simulink model "HCS_Sim_r9_final"  (R2023a)
settings: Solver=ode4  StartTime=0.0  StopTime=24  FixedStep=5e-3  RelTol=1e-3  EnableMultiTasking=on
libraries: simulink x26, simulink_extras x11, arduinolib x8, spspowerguiLib x1
(part 4 of 5)

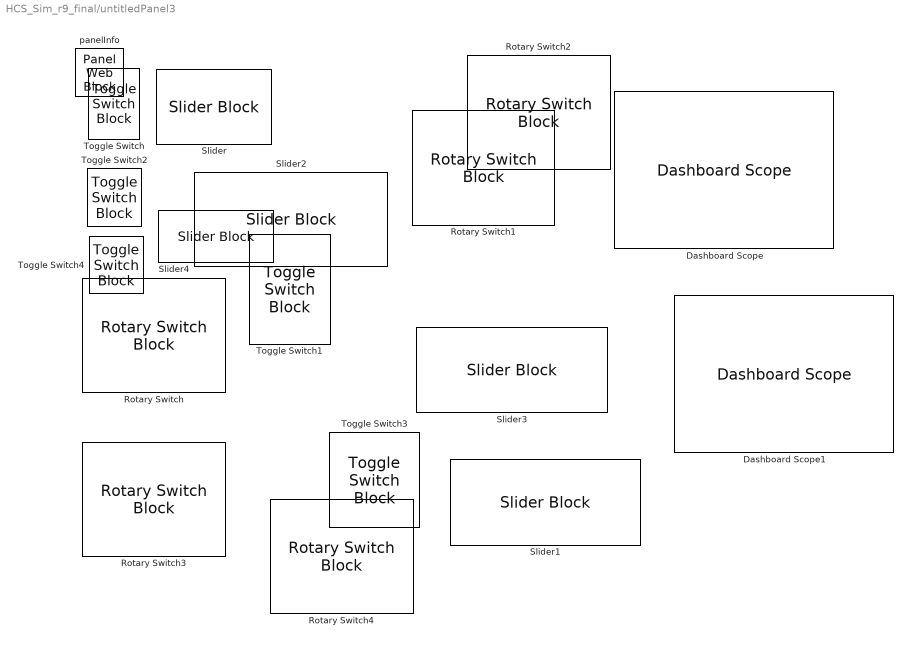
== system HCS_Sim_r9_final/untitledPanel3 ==
  Dashboard Scope : DashboardScope  Tag=HiddenForWebPanel  PanelInfo="{\"height\":377,\"left\":709,\"panelId\":\"panelId-5b2835c8-b6db-4cff-a750-dd4ee5f35628\",\"top\":424,\"type\":\"panelChild\",\"version\":\"2019b\",\"width\":535,\"zIndex\":1500032}"
  Dashboard Scope1 : DashboardScope  Tag=HiddenForWebPanel  PanelInfo="{\"height\":385,\"left\":705,\"panelId\":\"panelId-5b2835c8-b6db-4cff-a750-dd4ee5f35628\",\"top\":16,\"type\":\"panelChild\",\"version\":\"2019b\",\"width\":524,\"zIndex\":1500034}"
  Rotary Switch : RotarySwitchBlock  Tag=HiddenForWebPanel  PanelInfo="{\"height\":145,\"left\":20,\"panelId\":\"panelId-5b2835c8-b6db-4cff-a750-dd4ee5f35628\",\"top\":16,\"type\":\"panelChild\",\"version\":\"2019b\",\"width\":182,\"zIndex\":1500016}"
      settings: Values={{'>0', '1', '2', '3', '4'}, [0 1 2 3 4]}
      settings: AttributesFormatString=Hydrogren Level
  Rotary Switch1 : RotarySwitchBlock  Tag=HiddenForWebPanel  PanelInfo="{\"height\":145,\"left\":24,\"panelId\":\"panelId-5b2835c8-b6db-4cff-a750-dd4ee5f35628\",\"top\":177,\"type\":\"panelChild\",\"version\":\"2019b\",\"width\":182,\"zIndex\":1500014}"
      settings: Values={{'>0', '1', '2', '3', '4'}, [0 1 2 3 4]}
      settings: AttributesFormatString=Hydrogren Level
  Rotary Switch2 : RotarySwitchBlock  Tag=HiddenForWebPanel  PanelInfo="{\"height\":145,\"left\":24,\"panelId\":\"panelId-5b2835c8-b6db-4cff-a750-dd4ee5f35628\",\"top\":334,\"type\":\"panelChild\",\"version\":\"2019b\",\"width\":182,\"zIndex\":1500018}"
      settings: Values={{'>0', '1', '2', '3', '4'}, [0 1 2 3 4]}
      settings: AttributesFormatString=Hydrogren Level
  Rotary Switch3 : RotarySwitchBlock  Tag=HiddenForWebPanel  PanelInfo="{\"height\":145,\"left\":26,\"panelId\":\"panelId-5b2835c8-b6db-4cff-a750-dd4ee5f35628\",\"top\":492,\"type\":\"panelChild\",\"version\":\"2019b\",\"width\":182,\"zIndex\":1500020}"
      settings: Values={{'>0', '1', '2', '3', '4'}, [0 1 2 3 4]}
      settings: AttributesFormatString=Hydrogren Level
  Rotary Switch4 : RotarySwitchBlock  Tag=HiddenForWebPanel  PanelInfo="{\"height\":145,\"left\":33,\"panelId\":\"panelId-5b2835c8-b6db-4cff-a750-dd4ee5f35628\",\"top\":649,\"type\":\"panelChild\",\"version\":\"2019b\",\"width\":182,\"zIndex\":1500022}"
      settings: Values={{'>0', '1', '2', '3', '4'}, [0 1 2 3 4]}
      settings: AttributesFormatString=Hydrogren Level
  Slider : SliderBlock  Tag=HiddenForWebPanel  PanelInfo="{\"height\":135,\"left\":211,\"panelId\":\"panelId-5b2835c8-b6db-4cff-a750-dd4ee5f35628\",\"top\":22,\"type\":\"panelChild\",\"version\":\"2019b\",\"width\":253,\"zIndex\":1500008}"  ScaleMax=24
      settings: AttributesFormatString=Start Time
  Slider1 : SliderBlock  Tag=HiddenForWebPanel  PanelInfo="{\"height\":145,\"left\":217,\"panelId\":\"panelId-5b2835c8-b6db-4cff-a750-dd4ee5f35628\",\"top\":492,\"type\":\"panelChild\",\"version\":\"2019b\",\"width\":247,\"zIndex\":1500026}"  ScaleMax=24
      settings: AttributesFormatString=Start Time
  Slider2 : SliderBlock  Tag=HiddenForWebPanel  PanelInfo="{\"height\":145,\"left\":215,\"panelId\":\"panelId-5b2835c8-b6db-4cff-a750-dd4ee5f35628\",\"top\":177,\"type\":\"panelChild\",\"version\":\"2019b\",\"width\":236,\"zIndex\":1500036}"  ScaleMax=24  TickInterval=3
  Slider3 : SliderBlock  Tag=HiddenForWebPanel  PanelInfo="{\"height\":137,\"left\":217,\"panelId\":\"panelId-5b2835c8-b6db-4cff-a750-dd4ee5f35628\",\"top\":336,\"type\":\"panelChild\",\"version\":\"2019b\",\"width\":241,\"zIndex\":1500024}"  ScaleMax=24
      settings: AttributesFormatString=Start Time
  Slider4 : SliderBlock  Tag=HiddenForWebPanel  PanelInfo="{\"height\":133,\"left\":227,\"panelId\":\"panelId-5b2835c8-b6db-4cff-a750-dd4ee5f35628\",\"top\":654,\"type\":\"panelChild\",\"version\":\"2019b\",\"width\":242,\"zIndex\":1500012}"  ScaleMax=24
      settings: AttributesFormatString=Start Time
  Toggle Switch : ToggleSwitchBlock  Tag=HiddenForWebPanel  PanelInfo="{\"height\":140,\"left\":472,\"panelId\":\"panelId-5b2835c8-b6db-4cff-a750-dd4ee5f35628\",\"top\":11,\"type\":\"panelChild\",\"version\":\"2019b\",\"width\":131,\"zIndex\":1500002}"
      settings: Values={{'Off', 'On'}, [0 1]}
  Toggle Switch1 : ToggleSwitchBlock  Tag=HiddenForWebPanel  PanelInfo="{\"height\":129,\"left\":473,\"panelId\":\"panelId-5b2835c8-b6db-4cff-a750-dd4ee5f35628\",\"top\":160,\"type\":\"panelChild\",\"version\":\"2019b\",\"width\":130,\"zIndex\":1500028}"
      settings: Values={{'Off', 'On'}, [0 1]}
  Toggle Switch2 : ToggleSwitchBlock  Tag=HiddenForWebPanel  PanelInfo="{\"height\":142,\"left\":479,\"panelId\":\"panelId-5b2835c8-b6db-4cff-a750-dd4ee5f35628\",\"top\":468,\"type\":\"panelChild\",\"version\":\"2019b\",\"width\":133,\"zIndex\":1500004}"
      settings: Values={{'Off', 'On'}, [0 1]}
  Toggle Switch3 : ToggleSwitchBlock  Tag=HiddenForWebPanel  PanelInfo="{\"height\":155,\"left\":483,\"panelId\":\"panelId-5b2835c8-b6db-4cff-a750-dd4ee5f35628\",\"top\":624,\"type\":\"panelChild\",\"version\":\"2019b\",\"width\":140,\"zIndex\":1500030}"
      settings: Values={{'Off', 'On'}, [0 1]}
  Toggle Switch4 : ToggleSwitchBlock  Tag=HiddenForWebPanel  PanelInfo="{\"height\":148,\"left\":479,\"panelId\":\"panelId-5b2835c8-b6db-4cff-a750-dd4ee5f35628\",\"top\":301,\"type\":\"panelChild\",\"version\":\"2019b\",\"width\":126,\"zIndex\":1500006}"
      settings: Values={{'Off', 'On'}, [0 1]}
  panelInfo : PanelWebBlock  Tag=HiddenForWebPanel  PanelInfo="{\"compacted\":false,\"height\":812,\"isActiveTab\":true,\"left\":344,\"name\":\"Panel3\",\"panelId\":\"panelId-5b2835c8-b6db-4cff-a750-dd4ee5f35628\",\"tabIndex\":3,\"tabbedSetId\":\"tabbedSet1419519353\",\"top\":42,\"type\":\"panel\",\"version\":\"2019b\",\"visible\":true,\"width\":1334,\"zIndex\":1500006}"  PanelSnapshot=<binary blob, 125788 chars, not shown>  PanelBackground=data:image/png;base64,iVBORw0KGgoAAAANSUhEUgAAA9QAAAJiCAYAAAAmMIpYAAAAAXNSR0IArs4c6QAAAARnQU1BAACxjwv8YQUAAAAJcEhZcwAADsQAAA7EAZUrDhsAAE72SURBVHhe7d15tGZ5WR/636nh1Fw9NyBiCyIqaLyAEUQUUa8iOCBOBMc4haiEqwQ14sq9ioBTdCUKLr1CEgeUdRMjiDgQBQ0GEwcUBJRWBJFOC/RQ46mqU+fU/X33fp9zdr+eBtxBu4bPZ62nf8Pe73Tgn289+93vyoWuAQAAAH8nuxYjAAAA8HcgUAMAAMAMAjUAAADMIFADAADADAI1AAAAzCBQAwAAwAwCNQAAAMwgUAMAAMAMAjUAAADMIFADAADADAI1AAAAzCBQAwAAwAwCNQAA ...(+26696 chars)

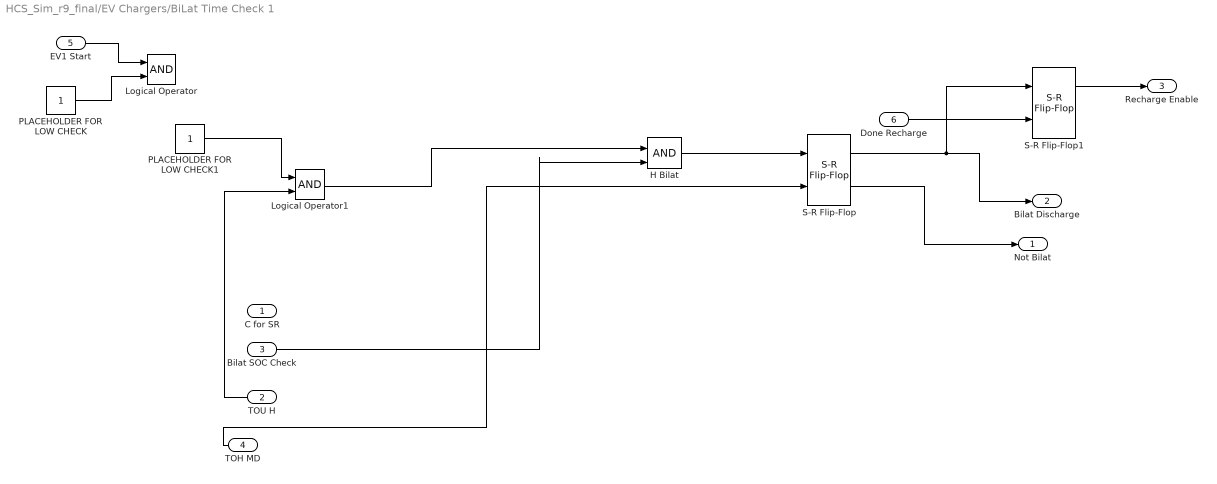
== system HCS_Sim_r9_final/EV Chargers/BiLat Time Check 1 ==
  C for SR : Inport
  TOU H : Inport  Port=2
  Bilat SOC Check : Inport  Port=3
  TOH MD : Inport  Port=4
  EV1 Start : Inport  Port=5
  Done Recharge : Inport  Port=6
  H Bilat : Logic  IconShape=distinctive  AllPortsSameDT=off  OutDataTypeStr=boolean
  Logical Operator : Logic  AllPortsSameDT=off  OutDataTypeStr=boolean
  Logical Operator1 : Logic  AllPortsSameDT=off  OutDataTypeStr=boolean
  PLACEHOLDER FOR LOW CHECK : Constant
  PLACEHOLDER FOR LOW CHECK1 : Constant
  S-R Flip-Flop : simulink_extras/Flip Flops/S-R Flip-Flop  initial_condition=0
  S-R Flip-Flop1 : simulink_extras/Flip Flops/S-R Flip-Flop  initial_condition=0
  Not Bilat : Outport
  Bilat Discharge : Outport  Port=2
  Recharge Enable : Outport  Port=3
  wires:
  TOH MD/1 -> S-R Flip-Flop/2
  Logical Operator1/1 -> H Bilat/1
  PLACEHOLDER FOR LOW CHECK1/1 -> Logical Operator1/1
  H Bilat/1 -> S-R Flip-Flop/1
  S-R Flip-Flop/1 -> S-R Flip-Flop1/1, Bilat Discharge/1
  S-R Flip-Flop/2 -> Not Bilat/1
  Bilat SOC Check/1 -> H Bilat/2
  TOU H/1 -> Logical Operator1/2
  PLACEHOLDER FOR LOW CHECK/1 -> Logical Operator/2
  EV1 Start/1 -> Logical Operator/1
  S-R Flip-Flop1/1 -> Recharge Enable/1
  Done Recharge/1 -> S-R Flip-Flop1/2

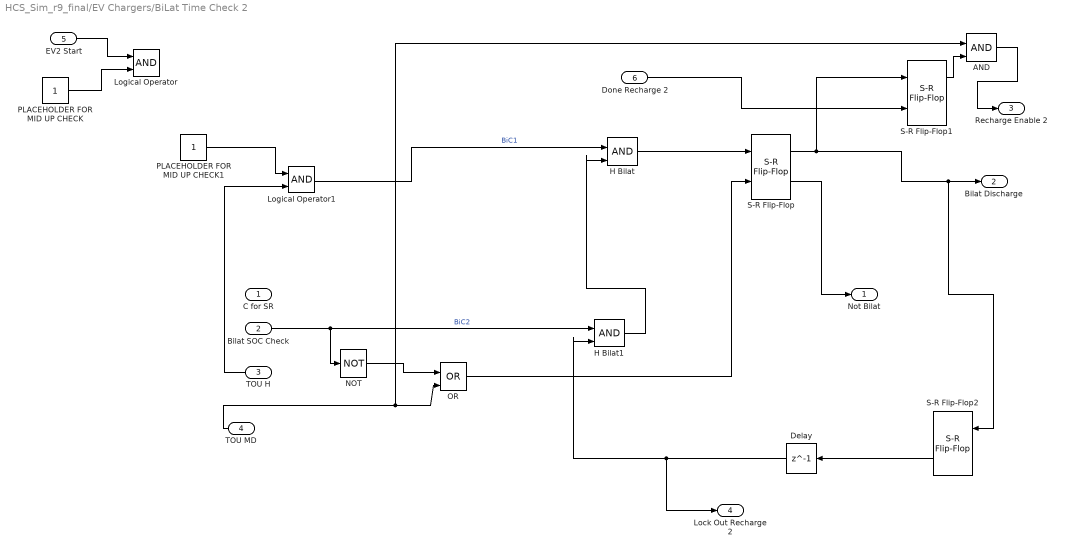
== system HCS_Sim_r9_final/EV Chargers/BiLat Time Check 2 ==
  C for SR : Inport
  Bilat SOC Check : Inport  Port=2
  TOU H : Inport  Port=3
  TOU MD : Inport  Port=4
  EV2 Start : Inport  Port=5
  Done Recharge 2 : Inport  Port=6
  AND : Logic  IconShape=distinctive  AllPortsSameDT=off  OutDataTypeStr=boolean
  Delay : Delay  DelayLength=1  InitialCondition=0
  H Bilat : Logic  IconShape=distinctive  AllPortsSameDT=off  OutDataTypeStr=boolean
  H Bilat1 : Logic  IconShape=distinctive  AllPortsSameDT=off  OutDataTypeStr=boolean
  Logical Operator : Logic  AllPortsSameDT=off  OutDataTypeStr=boolean
  Logical Operator1 : Logic  AllPortsSameDT=off  OutDataTypeStr=boolean
  NOT : Logic  Operator=NOT  IconShape=distinctive  AllPortsSameDT=off  OutDataTypeStr=boolean
  OR : Logic  Operator=OR  IconShape=distinctive  AllPortsSameDT=off  OutDataTypeStr=boolean
  PLACEHOLDER FOR MID UP CHECK : Constant
  PLACEHOLDER FOR MID UP CHECK1 : Constant
  S-R Flip-Flop : simulink_extras/Flip Flops/S-R Flip-Flop  initial_condition=0
  S-R Flip-Flop1 : simulink_extras/Flip Flops/S-R Flip-Flop  initial_condition=0
  S-R Flip-Flop2 : simulink_extras/Flip Flops/S-R Flip-Flop  initial_condition=0
  Not Bilat : Outport
  Bilat Discharge : Outport  Port=2
  Recharge Enable 2 : Outport  Port=3
  Lock Out Recharge 2 : Outport  Port=4
  wires:
  Logical Operator1/1 -> H Bilat/1  "BiC1"
  PLACEHOLDER FOR MID UP CHECK1/1 -> Logical Operator1/1
  S-R Flip-Flop/1 -> S-R Flip-Flop1/1, S-R Flip-Flop2/1, Bilat Discharge/1
  H Bilat/1 -> S-R Flip-Flop/1
  S-R Flip-Flop/2 -> Not Bilat/1
  Bilat SOC Check/1 -> H Bilat1/1, NOT/1  "BiC2"
  TOU H/1 -> Logical Operator1/2
  EV2 Start/1 -> Logical Operator/1
  PLACEHOLDER FOR MID UP CHECK/1 -> Logical Operator/2
  TOU MD/1 -> AND/1, OR/2
  Done Recharge 2/1 -> S-R Flip-Flop1/2
  AND/1 -> Recharge Enable 2/1
  OR/1 -> S-R Flip-Flop/2
  NOT/1 -> OR/1
  H Bilat1/1 -> H Bilat/2
  S-R Flip-Flop2/2 -> Delay/1
  Delay/1 -> Lock Out Recharge 2/1, H Bilat1/2
  S-R Flip-Flop1/1 -> AND/2

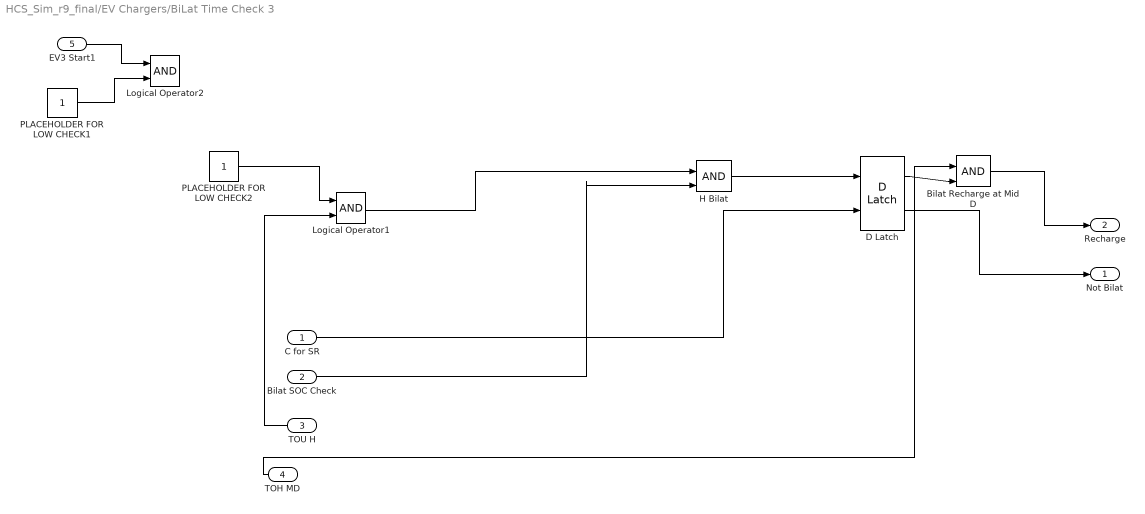
== system HCS_Sim_r9_final/EV Chargers/BiLat Time Check 3 ==
  C for SR : Inport
  Bilat SOC Check : Inport  Port=2
  TOU H : Inport  Port=3
  TOH MD : Inport  Port=4
  EV3 Start1 : Inport  Port=5
  Bilat Recharge at Mid D : Logic  IconShape=distinctive  AllPortsSameDT=off  OutDataTypeStr=boolean
  D Latch : simulink_extras/Flip Flops/D Latch
  H Bilat : Logic  IconShape=distinctive  AllPortsSameDT=off  OutDataTypeStr=boolean
  Logical Operator1 : Logic  AllPortsSameDT=off  OutDataTypeStr=boolean
  Logical Operator2 : Logic  AllPortsSameDT=off  OutDataTypeStr=boolean
  PLACEHOLDER FOR LOW CHECK1 : Constant
  PLACEHOLDER FOR LOW CHECK2 : Constant
  Not Bilat : Outport
  Recharge : Outport  Port=2
  wires:
  TOH MD/1 -> Bilat Recharge at Mid D/1
  Logical Operator1/1 -> H Bilat/1
  PLACEHOLDER FOR LOW CHECK2/1 -> Logical Operator1/1
  Bilat Recharge at Mid D/1 -> Recharge/1
  H Bilat/1 -> D Latch/1
  D Latch/1 -> Bilat Recharge at Mid D/2
  D Latch/2 -> Not Bilat/1
  C for SR/1 -> D Latch/2
  Bilat SOC Check/1 -> H Bilat/2
  TOU H/1 -> Logical Operator1/2
  EV3 Start1/1 -> Logical Operator2/1
  PLACEHOLDER FOR LOW CHECK1/1 -> Logical Operator2/2

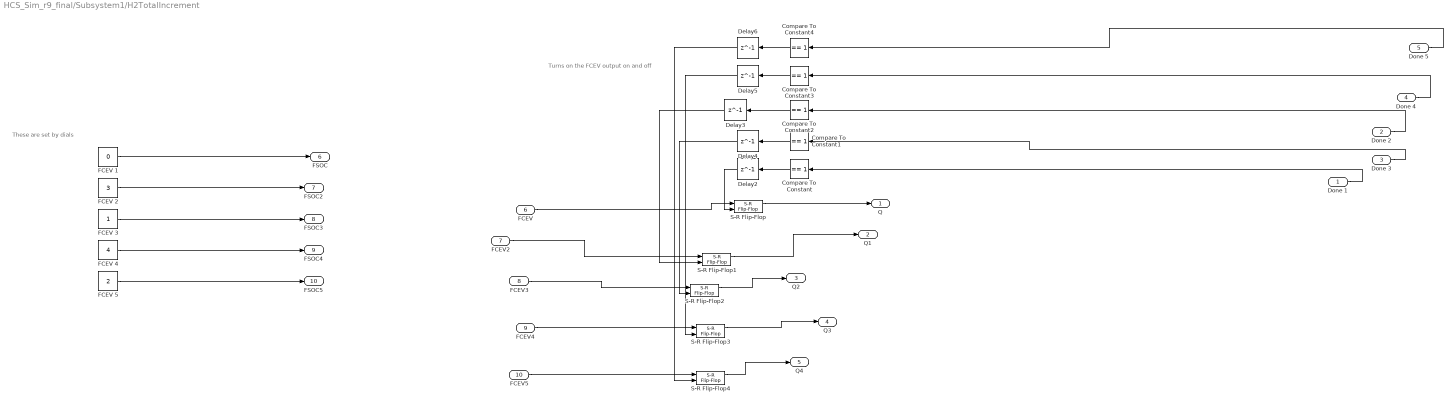
== system HCS_Sim_r9_final/Subsystem1/H2TotalIncrement ==
  note: Turns on the FCEV output
      | on and off
  note: These are set by dials
  Done 1 : Inport
  Done 2 : Inport  Port=2
  Done 3 : Inport  Port=3
  Done 4 : Inport  Port=4
  Done 5 : Inport  Port=5
  FCEV : Inport  Port=6
  FCEV2 : Inport  Port=7
  FCEV3 : Inport  Port=8
  FCEV4 : Inport  Port=9
  FCEV5 : Inport  Port=10
  Compare To Constant{,1..4} (5 alike) : simulink/Logic and Bit Operations/Compare To Constant  relop===  const=1  OutDataTypeStr=boolean
  Delay{2..6} (5 alike) : Delay  DelayLength=1  InitialCondition=0
  FCEV 1 : Constant  Value=0
  FCEV 2 : Constant  Value=3
  FCEV 3 : Constant
  FCEV 4 : Constant  Value=4
  FCEV 5 : Constant  Value=2
  S-R Flip-Flop{,1..4} (5 alike) : simulink_extras/Flip Flops/S-R Flip-Flop  initial_condition=0
  Q : Outport
  Q1 : Outport  Port=2
  Q2 : Outport  Port=3
  Q3 : Outport  Port=4
  Q4 : Outport  Port=5
  FSOC : Outport  Port=6
  FSOC2 : Outport  Port=7
  FSOC3 : Outport  Port=8
  FSOC4 : Outport  Port=9
  FSOC5 : Outport  Port=10
  wires:
  Done 5/1 -> Compare To Constant4/1
  Delay2/1 -> S-R Flip-Flop/2
  Delay4/1 -> S-R Flip-Flop2/2
  FCEV 3/1 -> FSOC3/1
  FCEV4/1 -> S-R Flip-Flop3/1
  FCEV 4/1 -> FSOC4/1
  Done 4/1 -> Compare To Constant3/1
  Delay6/1 -> S-R Flip-Flop4/2
  Compare To Constant4/1 -> Delay6/1
  Compare To Constant1/1 -> Delay4/1
  Compare To Constant3/1 -> Delay5/1
  Compare To Constant2/1 -> Delay3/1
  Compare To Constant/1 -> Delay2/1
  Delay3/1 -> S-R Flip-Flop1/2
  Delay5/1 -> S-R Flip-Flop3/2
  S-R Flip-Flop/1 -> Q/1
  S-R Flip-Flop4/1 -> Q4/1
  FCEV 5/1 -> FSOC5/1
  S-R Flip-Flop1/1 -> Q1/1
  FCEV5/1 -> S-R Flip-Flop4/1
  Done 1/1 -> Compare To Constant/1
  S-R Flip-Flop3/1 -> Q3/1
  Done 2/1 -> Compare To Constant2/1
  FCEV2/1 -> S-R Flip-Flop1/1
  S-R Flip-Flop2/1 -> Q2/1
  FCEV/1 -> S-R Flip-Flop/1
  FCEV 1/1 -> FSOC/1
  Done 3/1 -> Compare To Constant1/1
  FCEV 2/1 -> FSOC2/1
  FCEV3/1 -> S-R Flip-Flop2/1

== matlab function HCS_Sim_r9_final/EV Chargers/MATLAB Function1 ==
  data: ev1_bilat_OK output; ev2_bilat_OK output; ev3_bilat_OK output; soc_ev1 input; ev1_OK input; soc_ev2 input; ev2_OK input; soc_ev3 input; ev1_chargeBool output; ev2_chargeBool output; ev3_chargeBool output; ev3_OK input
  function [ev1_bilat_OK, ev2_bilat_OK, ev3_bilat_OK, ev1_chargeBool, ev2_chargeBool, ev3_chargeBool] = pctSOCCheck(soc_ev1, ev1_OK, soc_ev2, ev2_OK, soc_ev3, ev3_OK)
    bilatPartition = 90; % pct SOC
    fullCharge = 100; % pct SOC
    
    soc_ev_array = [soc_ev1, soc_ev2, soc_ev3]; % array of SOC for each EV
    ev_OK = [ev1_OK, ev2_OK, ev3_OK];
    ev_full = zeros(1, 3);
    ev_remaining = zeros(1, 3);
    ev_soc_AND = zeros(1, 3);
    bilat_OK = zeros(1, 3);
    chargeBool = zeros(1, 3);

    % computes the difference values (i.e., Pct of charge > 90% and Pct of
    % battery remaining)
    for i = 1:length(soc_ev_array)
        ev_amt = soc_ev_array(i) - bilatPartition;
        ev_remaining(i) = fullCharge - soc_ev_array(i);
        

        % (boolean) check if EV has charge >90%
        if ev_amt > 0
            ev_full(i) = 1;
        else 
            ev_full(i) = 0;
        end
        
        % (boolean) check if battery capacity remaining is > 2%
        if ev_remaining(i) > 2
            ev_soc_AND(i) = 1;
        else
            ev_soc_AND(i) = 0;
        end
        
        % (boolean) If EV is over 90% charged AND more than 2% of total
        % battery capacity is NOT available (battery SOC is > 98%),
        % initiate Bilateral Charging Available signal
        if (ev_full(i) == 1) && (ev_soc_AND(i) == 0)
            bilat_OK(i) = 1; % bilateral charging is available
        else
            bilat_OK(i) = 0; % bilateral charging is not available
        end
        
        % (boolean) If ev_OK signal is detected (i.e., EV is connected to
        % EVSE) AND >2% of total battery is remaining, output chargeBool
        % chargeBool is a boolean that communicates whether or not an EV is
        % maxxed out in charge
        if (ev_OK(i) == 1) && (ev_soc_AND(i) == 1)
            chargeBool(i) = 1; %% ON if EV is connected and SOC is <98%
        else
            chargeBool(i) = 0;
        end

    end

    
    ev1_bilat_OK = bilat_OK(1);
    ev2_bilat_OK = bilat_OK(2);
    ev3_bilat_OK = bilat_OK(3);

    % ev1_full = ev_full(1);
    % ev2_full = ev_full(2);
    % ev3_full = ev_full(3); % used for debugging earlier

    % ev1_remaining = ev_remaining(1);
    % ev2_remaining = ev_remaining(2);
    % ev3_remaining = ev_remaining(3); % used for debugging earlier

    ev1_chargeBool = chargeBool(1);
    ev2_chargeBool = chargeBool(2);
    ev3_chargeBool = chargeBool(3); 

end

== matlab function HCS_Sim_r9_final/EV Chargers/MATLAB Function2 ==
  data: ev_start_signal input; bilat_OK input; chargeEnable output; tou_int input; bilatEnable output; maxCharge input; incrementEV output
function [chargeEnable, bilatEnable, incrementEV] = ev_charge_ctrl(ev_start_signal, bilat_OK, tou_int, maxCharge)
    s = 0;
    bilatEnable = 0;
    chargeEnable = 0;
    
    % loop only starts if TOU is ON PEAK and if an EV has been detected by
    % the EVSE
    while (tou_int == 4 && ev_start_signal == 1)
        if bilat_OK == 1
            bilatEnable = 1; % bilateral discharge enabled
        else
            bilatEnable = 0; % bilateral discharge disabled
        end
        
        if (ev_start_signal == 1) && (bilat_OK == 0)
            chargeEnable = 1; % car is connected and battery is > 90% charged AND more then 2% of total capacity is available
        else
            chargeEnable = 0;
        end
    end
    
    % if bilat_OK == 0 (EV not ready for V2G) the vehicle is OK to charge
    % but is not currently, enable charging
    if (chargeEnable == 0) && (bilatEnable == 0)
        chargeEnable = 1;
    end

    % if bilateral charging is OFF and battery is NOT at max capacity, increment the EV
    % charge 
    if bilatEnable == 0 && maxCharge == 1
        incrementEV = 1; % increment charge
    else
        incrementEV = 0;
    end

    % if (chargeEnable == 1 && bilatEnable == 0) && maxCharge == 1
    %     rechargeTrig = 1; % send signal to controller to switch from Off/Bidirectional state to recharge mode
    % else
    %     rechargeTrig = 0;
    % end
    % 

end

== matlab function HCS_Sim_r9_final/Flywheel/SoC-kWh Conversion (Flywheel) ==
  data: flywheel_soc_in input; kwh_g2fly output; kwh_fly2g output; flywheel_soc_out input
function [kwh_g2fly, kwh_fly2g] = flywheel_soc_kwh_convert(flywheel_soc_in, flywheel_soc_out)
% Function purpose is to take EV SoC and compute kWh consumed
% kwh_g2v output is a 1x3 array logging kWh drawn from the grid
% kwh_v2g output is 1x3 array logging kWh sold back to grid
flywheel_kwh_capacity = 130; % kWh (full flywheel capacity)

persistent kwh_g2fly_total kwh_fly2g_total
if isempty(kwh_g2fly_total)
    kwh_g2fly_total = 0;
end

if isempty(kwh_fly2g_total)
    kwh_fly2g_total = 0;
end


kwh_g2fly_total = flywheel_kwh_capacity * flywheel_soc_in;
kwh_fly2g_total = (flywheel_kwh_capacity * flywheel_soc_out) * 0.95; % multiply by 0.90 to approximate losses



kwh_g2fly = kwh_g2fly_total;
kwh_fly2g = kwh_fly2g_total;

== matlab function HCS_Sim_r9_final/MATLAB Function2 ==
  data: time input; vehConnected input; batteryCapacity output; vehicleID input; batteryCapacity input; ev_SOC input; connectorIn input; connectorOut input; ev_SOC_new output
function [batteryCapacity, ev_SOC_new] = vehicleSpecs(time, vehConnected, vehicleID, batteryCapacity, ev_SOC, connectorIn, connectorOut)
% vehicleID (integer): value that specifies the car number connected
% batteryCapacity: Max capacity of vehicle battery (in kWh)
% ev_SOC: Cummulative SOC of connected vehicle 
% connectorIn: time connector is inserted into charge port
% connectorOut: time connector is removed from charge port
batteryCapacity = 1;
ev_SOC_new = 1;

end

== matlab function HCS_Sim_r9_final/Flywheel/Flywheel Function (New) ==
  data: flywheel_soc input; flywheel_soc_new output; scaling input; tou input; flywheelMode output; incrementFlywheel output; fw_soc_in input; fw_soc_out input; new_soc_in output; new_soc_out output; flywheel_rpm output; flywheelState output; manualDischarge input
function [flywheel_soc_new, flywheelMode, incrementFlywheel, new_soc_in, new_soc_out, flywheel_rpm, flywheelState] = flywheel(flywheel_soc, scaling, tou, fw_soc_in, fw_soc_out, manualDischarge)
% tou: time of use integer
%   [1] off peak
%   [2] mid peak low/down
%   [3] mid peak high
%   [4] on peak
%   [5] null
% fwChargeStep: increment fw up or down
% fwCapacity: static value
% flywheel_soc:  current state of charge

fwCapacity = 130; % kwh
fwChargePerHr = 65 * scaling * 0.01;
maxRPM = 45;
flywheel_rpm = maxRPM * flywheel_soc;
%flywheel_soc_new = flywheel_soc;

if manualDischarge == 0
    if (tou == 1) && (flywheel_soc < 0.99) % off peak OR mid peak low, and SOC <= 98%
            incrementFlywheel = fwChargePerHr / fwCapacity; % charge
            flywheel_soc_new = flywheel_soc + incrementFlywheel;
            new_soc_in = fw_soc_in + incrementFlywheel; % track SoC % change INTO flywheel
            new_soc_out = fw_soc_out; % track SoC % change OUT flywheel (no change if charging mode)
            % Indicate charging state (Arduino interfacing)
            flywheelMode = 1;
            flywheelState = 1;
        % elseif (flywheel_soc > 0.99 && flywheel_soc < 1.00)
            %incrementFlywheel = 
    elseif (tou == 4) && (flywheel_soc > 0) % discharge when on peak
        incrementFlywheel = -fwChargePerHr / fwCapacity;
        flywheel_soc_new = flywheel_soc + incrementFlywheel;
        new_soc_in = fw_soc_in; 
        new_soc_out = fw_soc_out + -(incrementFlywheel);
        % Indicate discharging state (Arduino interfacing)
        flywheelMode = 1; % discharging
        flywheelState = -1;
    elseif (tou == 2) && (flywheel_soc > 0) % discharge when on peak
        incrementFlywheel = -fwChargePerHr / fwCapacity;
        flywheel_soc_new = flywheel_soc + incrementFlywheel;
        new_soc_in = fw_soc_in; 
        new_soc_out = fw_soc_out + -(incrementFlywheel);
        % Indicate discharging state (Arduino interfacing)
        flywheelMode = 1; % discharging
        flywheelState = -1;
    else
        incrementFlywheel = 0;
        flywheel_soc_new = flywheel_soc + incrementFlywheel;
        new_soc_in = fw_soc_in;
        new_soc_out = fw_soc_out;
        % Indicate idle/conservational state (Arduino interfacing)
        flywheelMode = 0;
        flywheelState = 0;
    end
else
    incrementFlywheel = -fwChargePerHr / fwCapacity;
    flywheel_soc_new = flywheel_soc + incrementFlywheel;
    new_soc_in = fw_soc_in; 
    new_soc_out = fw_soc_out + -(incrementFlywheel);
    % Indicate discharging state (Arduino interfacing)
    flywheelMode = 1; % discharging
    flywheelState = -1;
end
